simulink model "SWC_CGW_type"  (R2021b)
settings: Solver=FixedStepDiscrete  StartTime=0.0  StopTime=10.0  RelTol=1e-3
settings Model: DataDictionary=APPTypes.sldd  Creator=FVT23010  LastModifiedBy=FVT23010
settings DataIOCC: SaveFormat=StructureWithTime
settings OptimizationCC: DefaultParameterBehavior=Inlined  EnhancedBackFolding=on  PassReuseOutputArgsAs=Individual arguments  ZeroExternalMemoryAtStartup=off  ZeroInternalMemoryAtStartup=off  OptimizeBlockOrder=speed  DifferentSizesBufferReuse=on  OptimizationCustomize=off  EfficientTunableParamExpr=on
settings DebuggingCC: ParameterTunabilityLossMsg=error
settings HardwareCC: ProdBitPerPointer=32  ProdBitPerSizeT=32  ProdBitPerPtrDiffT=32  ProdLargestAtomicInteger=Long  ProdLargestAtomicFloat=Double  ProdWordSize=32  ProdLongLongMode=on  ProdHWDeviceType=ARM Compatible->ARM Cortex-M
settings ModelReferenceCC: ModelReferenceNumInstancesAllowed=Single
settings SFSimCC: MATLABDynamicMemAlloc=off
settings RTWCC: Description=AUTOSAR  SystemTargetFile=autosar.tlc  GenCodeOnly=on  TemplateMakefile=ert_default_tmf  PortableWordSizes=on
settings CodeAppCC: ForceParamTrailComments=on  IgnoreCustomStorageClasses=off  OperatorAnnotations=on  SimulinkDataObjDesc=on  SFDataObjDesc=on  InsertBlockDesc=on
settings STFCustomTargetCC: TargetLangStandard=C99 (ISO)  MultiwordLength=256  ParMdlRefBuildCompliant=on  CompOptLevelCompliant=on  IncludeMdlTerminateFcn=off  CombineOutputUpdateFcns=on  SuppressErrorStatus=on  ERTCustomFileBanners=on  SupportNonFinite=off  SupportComplex=off  SupportContinuousTime=off  SupportNonInlinedSFcns=off  RemoveResetFunc=on  MATLABClassNameForMDSCustomization=Simulink.SoftwareTarget.ERTCustomization  AutosarCompliant=on  GRTInterface=off  UseToolchainInfoCompliant=on  LookupTableObjectStructAxisOrder=2,1,3,4,...  LUTObjectStructOrderEvenSpacing=Size,Table,Breakpoints  SystemTargetFile=autosar.tlc
settings ERTTargetCC: TargetLangStandard=C99 (ISO)  ConcurrentExecutionCompliant=off  IncludeMdlTerminateFcn=off  SuppressErrorStatus=on  SupportNonFinite=off  SupportComplex=off  ModelStepFunctionPrototypeControlCompliant=off  CPPClassGenCompliant=off  AutosarCompliant=on  LookupTableObjectStructAxisOrder=2,1,3,4,...  LUTObjectStructOrderEvenSpacing=Size,Table,Breakpoints  GenerateASAP2=on  InlinedParameterPlacement=NonHierarchical  ERTCustomFileTemplate=example_file_process.tlc  ConvertIfToSwitch=off  SuppressUnreachableDefaultCases=off  BooleanTrueId=true_MatlabRTW  BooleanFalseId=false_MatlabRTW

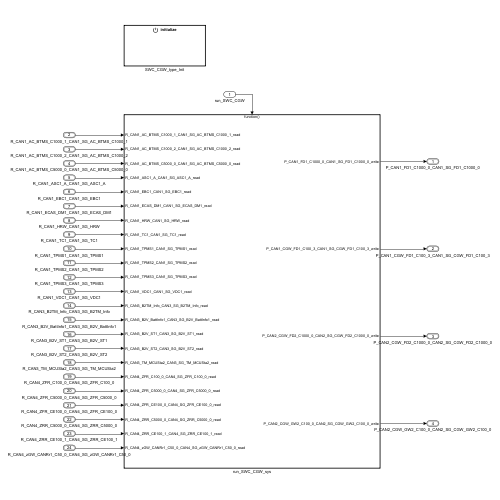
[thumbnail: Simulink's stored preview of the top-level diagram]
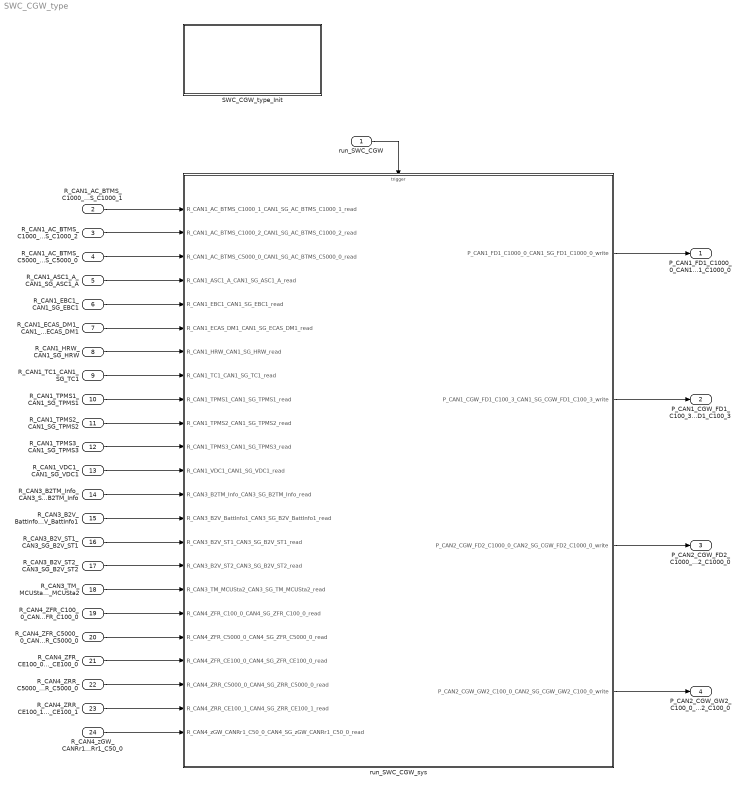
== system SWC_CGW_type ==
  run_SWC_CGW : Inport  OutputFunctionCall=on
  R_CAN1_AC_BTMS_C1000_1_CAN1_SG_AC_BTMS_C1000_1 : Inport  Port=2  OutDataTypeStr=Bus: DT_CAN1_SG_AC_BTMS_C1000_1  PortDimensions=1  BusOutputAsStruct=on
  R_CAN1_AC_BTMS_C1000_2_CAN1_SG_AC_BTMS_C1000_2 : Inport  Port=3  OutDataTypeStr=Bus: DT_CAN1_SG_AC_BTMS_C1000_2  PortDimensions=1  BusOutputAsStruct=on
  R_CAN1_AC_BTMS_C5000_0_CAN1_SG_AC_BTMS_C5000_0 : Inport  Port=4  OutDataTypeStr=Bus: DT_CAN1_SG_AC_BTMS_C5000_0  PortDimensions=1  BusOutputAsStruct=on
  R_CAN1_ASC1_A_CAN1_SG_ASC1_A : Inport  Port=5  OutDataTypeStr=Bus: DT_CAN1_SG_ASC1_A  PortDimensions=1  BusOutputAsStruct=on
  R_CAN1_EBC1_CAN1_SG_EBC1 : Inport  Port=6  OutDataTypeStr=Bus: DT_CAN1_SG_EBC1  PortDimensions=1  BusOutputAsStruct=on
  R_CAN1_ECAS_DM1_CAN1_SG_ECAS_DM1 : Inport  Port=7  OutDataTypeStr=Bus: DT_CAN1_SG_ECAS_DM1  PortDimensions=1  BusOutputAsStruct=on
  R_CAN1_HRW_CAN1_SG_HRW : Inport  Port=8  OutDataTypeStr=Bus: DT_CAN1_SG_HRW  PortDimensions=1  BusOutputAsStruct=on
  R_CAN1_TC1_CAN1_SG_TC1 : Inport  Port=9  OutDataTypeStr=Bus: DT_CAN1_SG_TC1  PortDimensions=1  BusOutputAsStruct=on
  R_CAN1_TPMS1_CAN1_SG_TPMS1 : Inport  Port=10  OutDataTypeStr=Bus: DT_CAN1_SG_TPMS1  PortDimensions=1  BusOutputAsStruct=on
  R_CAN1_TPMS2_CAN1_SG_TPMS2 : Inport  Port=11  OutDataTypeStr=Bus: DT_CAN1_SG_TPMS2  PortDimensions=1  BusOutputAsStruct=on
  R_CAN1_TPMS3_CAN1_SG_TPMS3 : Inport  Port=12  OutDataTypeStr=Bus: DT_CAN1_SG_TPMS3  PortDimensions=1  BusOutputAsStruct=on
  R_CAN1_VDC1_CAN1_SG_VDC1 : Inport  Port=13  OutDataTypeStr=Bus: DT_CAN1_SG_VDC1  PortDimensions=1  BusOutputAsStruct=on
  R_CAN3_B2TM_Info_CAN3_SG_B2TM_Info : Inport  Port=14  OutDataTypeStr=Bus: DT_CAN3_SG_B2TM_Info  PortDimensions=1  BusOutputAsStruct=on
  R_CAN3_B2V_BattInfo1_CAN3_SG_B2V_BattInfo1 : Inport  Port=15  OutDataTypeStr=Bus: DT_CAN3_SG_B2V_BattInfo1  PortDimensions=1  BusOutputAsStruct=on
  R_CAN3_B2V_ST1_CAN3_SG_B2V_ST1 : Inport  Port=16  OutDataTypeStr=Bus: DT_CAN3_SG_B2V_ST1  PortDimensions=1  BusOutputAsStruct=on
  R_CAN3_B2V_ST2_CAN3_SG_B2V_ST2 : Inport  Port=17  OutDataTypeStr=Bus: DT_CAN3_SG_B2V_ST2  PortDimensions=1  BusOutputAsStruct=on
  R_CAN3_TM_MCUSta2_CAN3_SG_TM_MCUSta2 : Inport  Port=18  OutDataTypeStr=Bus: DT_CAN3_SG_TM_MCUSta2  PortDimensions=1  BusOutputAsStruct=on
  R_CAN4_ZFR_C100_0_CAN4_SG_ZFR_C100_0 : Inport  Port=19  OutDataTypeStr=Bus: DT_CAN4_SG_ZFR_C100_0  PortDimensions=1  BusOutputAsStruct=on
  R_CAN4_ZFR_C5000_0_CAN4_SG_ZFR_C5000_0 : Inport  Port=20  OutDataTypeStr=Bus: DT_CAN4_SG_ZFR_C5000_0  PortDimensions=1  BusOutputAsStruct=on
  R_CAN4_ZFR_CE100_0_CAN4_SG_ZFR_CE100_0 : Inport  Port=21  OutDataTypeStr=Bus: DT_CAN4_SG_ZFR_CE100_0  PortDimensions=1  BusOutputAsStruct=on
  R_CAN4_ZRR_C5000_0_CAN4_SG_ZRR_C5000_0 : Inport  Port=22  OutDataTypeStr=Bus: DT_CAN4_SG_ZRR_C5000_0  PortDimensions=1  BusOutputAsStruct=on
  R_CAN4_ZRR_CE100_1_CAN4_SG_ZRR_CE100_1 : Inport  Port=23  OutDataTypeStr=Bus: DT_CAN4_SG_ZRR_CE100_1  PortDimensions=1  BusOutputAsStruct=on
  R_CAN4_zGW_CANRr1_C50_0_CAN4_SG_zGW_CANRr1_C50_0 : Inport  Port=24  OutDataTypeStr=Bus: DT_CAN4_SG_zGW_CANRr1_C50_0  PortDimensions=1  BusOutputAsStruct=on
  SWC_CGW_type_Init : Subsystem
  run_SWC_CGW_sys : Subsystem
  P_CAN1_FD1_C1000_0_CAN1_SG_FD1_C1000_0 : Outport  OutDataTypeStr=Bus: DT_CAN1_SG_FD1_C1000_0  PortDimensions=1  BusOutputAsStruct=on
  P_CAN1_CGW_FD1_C100_3_CAN1_SG_CGW_FD1_C100_3 : Outport  Port=2  OutDataTypeStr=Bus: DT_CAN1_SG_CGW_FD1_C100_3  PortDimensions=1  BusOutputAsStruct=on
  P_CAN2_CGW_FD2_C1000_0_CAN2_SG_CGW_FD2_C1000_0 : Outport  Port=3  OutDataTypeStr=Bus: DT_CAN2_SG_CGW_FD2_C1000_0  PortDimensions=1  BusOutputAsStruct=on
  P_CAN2_CGW_GW2_C100_0_CAN2_SG_CGW_GW2_C100_0 : Outport  Port=4  OutDataTypeStr=Bus: DT_CAN2_SG_CGW_GW2_C100_0  PortDimensions=1  BusOutputAsStruct=on
  wires:
  R_CAN1_AC_BTMS_C1000_1_CAN1_SG_AC_BTMS_C1000_1/1 -> run_SWC_CGW_sys/1(R_CAN1_AC_BTMS_C1000_1_CAN1_SG_AC_BTMS_C1000_1_read)
  R_CAN1_AC_BTMS_C1000_2_CAN1_SG_AC_BTMS_C1000_2/1 -> run_SWC_CGW_sys/2(R_CAN1_AC_BTMS_C1000_2_CAN1_SG_AC_BTMS_C1000_2_read)
  R_CAN1_AC_BTMS_C5000_0_CAN1_SG_AC_BTMS_C5000_0/1 -> run_SWC_CGW_sys/3(R_CAN1_AC_BTMS_C5000_0_CAN1_SG_AC_BTMS_C5000_0_read)
  R_CAN1_ASC1_A_CAN1_SG_ASC1_A/1 -> run_SWC_CGW_sys/4(R_CAN1_ASC1_A_CAN1_SG_ASC1_A_read)
  R_CAN1_EBC1_CAN1_SG_EBC1/1 -> run_SWC_CGW_sys/5(R_CAN1_EBC1_CAN1_SG_EBC1_read)
  R_CAN1_ECAS_DM1_CAN1_SG_ECAS_DM1/1 -> run_SWC_CGW_sys/6(R_CAN1_ECAS_DM1_CAN1_SG_ECAS_DM1_read)
  R_CAN1_HRW_CAN1_SG_HRW/1 -> run_SWC_CGW_sys/7(R_CAN1_HRW_CAN1_SG_HRW_read)
  R_CAN1_TC1_CAN1_SG_TC1/1 -> run_SWC_CGW_sys/8(R_CAN1_TC1_CAN1_SG_TC1_read)
  R_CAN1_TPMS1_CAN1_SG_TPMS1/1 -> run_SWC_CGW_sys/9(R_CAN1_TPMS1_CAN1_SG_TPMS1_read)
  R_CAN1_TPMS2_CAN1_SG_TPMS2/1 -> run_SWC_CGW_sys/10(R_CAN1_TPMS2_CAN1_SG_TPMS2_read)
  R_CAN1_TPMS3_CAN1_SG_TPMS3/1 -> run_SWC_CGW_sys/11(R_CAN1_TPMS3_CAN1_SG_TPMS3_read)
  R_CAN1_VDC1_CAN1_SG_VDC1/1 -> run_SWC_CGW_sys/12(R_CAN1_VDC1_CAN1_SG_VDC1_read)
  R_CAN3_B2TM_Info_CAN3_SG_B2TM_Info/1 -> run_SWC_CGW_sys/13(R_CAN3_B2TM_Info_CAN3_SG_B2TM_Info_read)
  R_CAN3_B2V_BattInfo1_CAN3_SG_B2V_BattInfo1/1 -> run_SWC_CGW_sys/14(R_CAN3_B2V_BattInfo1_CAN3_SG_B2V_BattInfo1_read)
  R_CAN3_B2V_ST1_CAN3_SG_B2V_ST1/1 -> run_SWC_CGW_sys/15(R_CAN3_B2V_ST1_CAN3_SG_B2V_ST1_read)
  R_CAN3_B2V_ST2_CAN3_SG_B2V_ST2/1 -> run_SWC_CGW_sys/16(R_CAN3_B2V_ST2_CAN3_SG_B2V_ST2_read)
  R_CAN3_TM_MCUSta2_CAN3_SG_TM_MCUSta2/1 -> run_SWC_CGW_sys/17(R_CAN3_TM_MCUSta2_CAN3_SG_TM_MCUSta2_read)
  R_CAN4_ZFR_C100_0_CAN4_SG_ZFR_C100_0/1 -> run_SWC_CGW_sys/18(R_CAN4_ZFR_C100_0_CAN4_SG_ZFR_C100_0_read)
  R_CAN4_ZFR_C5000_0_CAN4_SG_ZFR_C5000_0/1 -> run_SWC_CGW_sys/19(R_CAN4_ZFR_C5000_0_CAN4_SG_ZFR_C5000_0_read)
  R_CAN4_ZFR_CE100_0_CAN4_SG_ZFR_CE100_0/1 -> run_SWC_CGW_sys/20(R_CAN4_ZFR_CE100_0_CAN4_SG_ZFR_CE100_0_read)
  R_CAN4_ZRR_C5000_0_CAN4_SG_ZRR_C5000_0/1 -> run_SWC_CGW_sys/21(R_CAN4_ZRR_C5000_0_CAN4_SG_ZRR_C5000_0_read)
  R_CAN4_ZRR_CE100_1_CAN4_SG_ZRR_CE100_1/1 -> run_SWC_CGW_sys/22(R_CAN4_ZRR_CE100_1_CAN4_SG_ZRR_CE100_1_read)
  R_CAN4_zGW_CANRr1_C50_0_CAN4_SG_zGW_CANRr1_C50_0/1 -> run_SWC_CGW_sys/23(R_CAN4_zGW_CANRr1_C50_0_CAN4_SG_zGW_CANRr1_C50_0_read)
  run_SWC_CGW_sys/1(P_CAN1_FD1_C1000_0_CAN1_SG_FD1_C1000_0_write) -> P_CAN1_FD1_C1000_0_CAN1_SG_FD1_C1000_0/1
  run_SWC_CGW_sys/2(P_CAN1_CGW_FD1_C100_3_CAN1_SG_CGW_FD1_C100_3_write) -> P_CAN1_CGW_FD1_C100_3_CAN1_SG_CGW_FD1_C100_3/1
  run_SWC_CGW_sys/3(P_CAN2_CGW_FD2_C1000_0_CAN2_SG_CGW_FD2_C1000_0_write) -> P_CAN2_CGW_FD2_C1000_0_CAN2_SG_CGW_FD2_C1000_0/1
  run_SWC_CGW_sys/4(P_CAN2_CGW_GW2_C100_0_CAN2_SG_CGW_GW2_C100_0_write) -> P_CAN2_CGW_GW2_C100_0_CAN2_SG_CGW_GW2_C100_0/1
  run_SWC_CGW/1 -> run_SWC_CGW_sys/Trigger

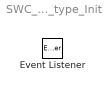
== system SWC_CGW_type/SWC_CGW_type_Init ==
  Event Listener : EventListener  EventName=reset

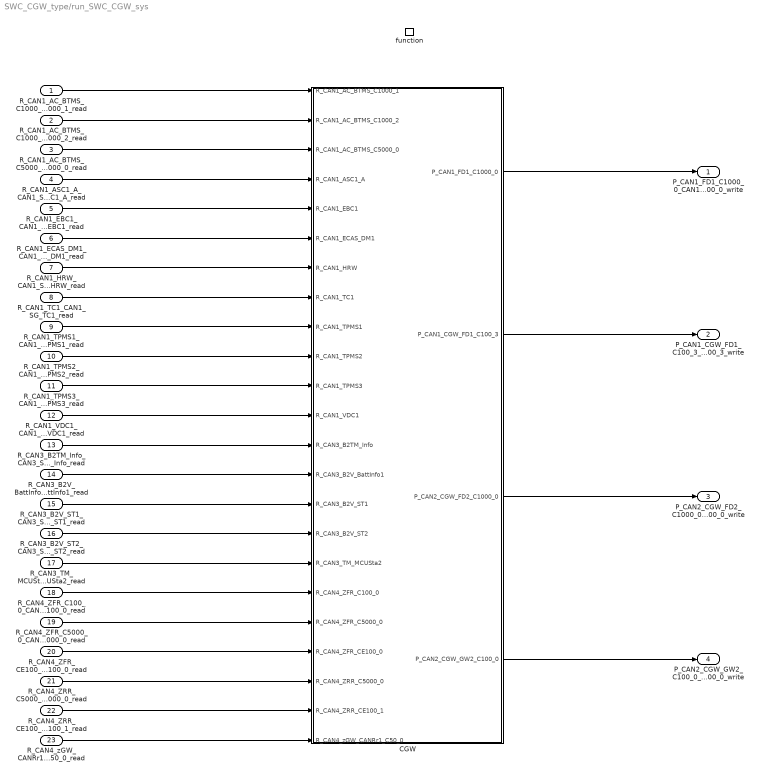
== system SWC_CGW_type/run_SWC_CGW_sys ==
  R_CAN1_AC_BTMS_C1000_1_CAN1_SG_AC_BTMS_C1000_1_read : Inport
  R_CAN1_AC_BTMS_C1000_2_CAN1_SG_AC_BTMS_C1000_2_read : Inport  Port=2
  R_CAN1_AC_BTMS_C5000_0_CAN1_SG_AC_BTMS_C5000_0_read : Inport  Port=3
  R_CAN1_ASC1_A_CAN1_SG_ASC1_A_read : Inport  Port=4
  R_CAN1_EBC1_CAN1_SG_EBC1_read : Inport  Port=5
  R_CAN1_ECAS_DM1_CAN1_SG_ECAS_DM1_read : Inport  Port=6
  R_CAN1_HRW_CAN1_SG_HRW_read : Inport  Port=7
  R_CAN1_TC1_CAN1_SG_TC1_read : Inport  Port=8
  R_CAN1_TPMS1_CAN1_SG_TPMS1_read : Inport  Port=9
  R_CAN1_TPMS2_CAN1_SG_TPMS2_read : Inport  Port=10
  R_CAN1_TPMS3_CAN1_SG_TPMS3_read : Inport  Port=11
  R_CAN1_VDC1_CAN1_SG_VDC1_read : Inport  Port=12
  R_CAN3_B2TM_Info_CAN3_SG_B2TM_Info_read : Inport  Port=13
  R_CAN3_B2V_BattInfo1_CAN3_SG_B2V_BattInfo1_read : Inport  Port=14
  R_CAN3_B2V_ST1_CAN3_SG_B2V_ST1_read : Inport  Port=15
  R_CAN3_B2V_ST2_CAN3_SG_B2V_ST2_read : Inport  Port=16
  R_CAN3_TM_MCUSta2_CAN3_SG_TM_MCUSta2_read : Inport  Port=17
  R_CAN4_ZFR_C100_0_CAN4_SG_ZFR_C100_0_read : Inport  Port=18
  R_CAN4_ZFR_C5000_0_CAN4_SG_ZFR_C5000_0_read : Inport  Port=19
  R_CAN4_ZFR_CE100_0_CAN4_SG_ZFR_CE100_0_read : Inport  Port=20
  R_CAN4_ZRR_C5000_0_CAN4_SG_ZRR_C5000_0_read : Inport  Port=21
  R_CAN4_ZRR_CE100_1_CAN4_SG_ZRR_CE100_1_read : Inport  Port=22
  R_CAN4_zGW_CANRr1_C50_0_CAN4_SG_zGW_CANRr1_C50_0_read : Inport  Port=23
  function : TriggerPort  TriggerType=function-call  VariantControl=(inherit)
  CGW : Subsystem
  P_CAN1_FD1_C1000_0_CAN1_SG_FD1_C1000_0_write : Outport
  P_CAN1_CGW_FD1_C100_3_CAN1_SG_CGW_FD1_C100_3_write : Outport  Port=2
  P_CAN2_CGW_FD2_C1000_0_CAN2_SG_CGW_FD2_C1000_0_write : Outport  Port=3
  P_CAN2_CGW_GW2_C100_0_CAN2_SG_CGW_GW2_C100_0_write : Outport  Port=4
  wires:
  R_CAN3_TM_MCUSta2_CAN3_SG_TM_MCUSta2_read/1 -> CGW/17(R_CAN3_TM_MCUSta2)
  R_CAN3_B2V_ST1_CAN3_SG_B2V_ST1_read/1 -> CGW/15(R_CAN3_B2V_ST1)
  R_CAN3_B2V_ST2_CAN3_SG_B2V_ST2_read/1 -> CGW/16(R_CAN3_B2V_ST2)
  R_CAN4_ZFR_C100_0_CAN4_SG_ZFR_C100_0_read/1 -> CGW/18(R_CAN4_ZFR_C100_0)
  R_CAN4_ZFR_C5000_0_CAN4_SG_ZFR_C5000_0_read/1 -> CGW/19(R_CAN4_ZFR_C5000_0)
  R_CAN3_B2TM_Info_CAN3_SG_B2TM_Info_read/1 -> CGW/13(R_CAN3_B2TM_Info)
  R_CAN3_B2V_BattInfo1_CAN3_SG_B2V_BattInfo1_read/1 -> CGW/14(R_CAN3_B2V_BattInfo1)
  R_CAN4_ZFR_CE100_0_CAN4_SG_ZFR_CE100_0_read/1 -> CGW/20(R_CAN4_ZFR_CE100_0)
  R_CAN4_ZRR_C5000_0_CAN4_SG_ZRR_C5000_0_read/1 -> CGW/21(R_CAN4_ZRR_C5000_0)
  R_CAN1_VDC1_CAN1_SG_VDC1_read/1 -> CGW/12(R_CAN1_VDC1)
  R_CAN4_ZRR_CE100_1_CAN4_SG_ZRR_CE100_1_read/1 -> CGW/22(R_CAN4_ZRR_CE100_1)
  R_CAN1_TPMS2_CAN1_SG_TPMS2_read/1 -> CGW/10(R_CAN1_TPMS2)
  R_CAN1_TPMS3_CAN1_SG_TPMS3_read/1 -> CGW/11(R_CAN1_TPMS3)
  R_CAN4_zGW_CANRr1_C50_0_CAN4_SG_zGW_CANRr1_C50_0_read/1 -> CGW/23(R_CAN4_zGW_CANRr1_C50_0)
  R_CAN1_TC1_CAN1_SG_TC1_read/1 -> CGW/8(R_CAN1_TC1)
  R_CAN1_TPMS1_CAN1_SG_TPMS1_read/1 -> CGW/9(R_CAN1_TPMS1)
  R_CAN1_HRW_CAN1_SG_HRW_read/1 -> CGW/7(R_CAN1_HRW)
  R_CAN1_EBC1_CAN1_SG_EBC1_read/1 -> CGW/5(R_CAN1_EBC1)
  R_CAN1_ECAS_DM1_CAN1_SG_ECAS_DM1_read/1 -> CGW/6(R_CAN1_ECAS_DM1)
  R_CAN1_AC_BTMS_C5000_0_CAN1_SG_AC_BTMS_C5000_0_read/1 -> CGW/3(R_CAN1_AC_BTMS_C5000_0)
  R_CAN1_ASC1_A_CAN1_SG_ASC1_A_read/1 -> CGW/4(R_CAN1_ASC1_A)
  R_CAN1_AC_BTMS_C1000_2_CAN1_SG_AC_BTMS_C1000_2_read/1 -> CGW/2(R_CAN1_AC_BTMS_C1000_2)
  R_CAN1_AC_BTMS_C1000_1_CAN1_SG_AC_BTMS_C1000_1_read/1 -> CGW/1(R_CAN1_AC_BTMS_C1000_1)
  CGW/1(P_CAN1_FD1_C1000_0) -> P_CAN1_FD1_C1000_0_CAN1_SG_FD1_C1000_0_write/1
  CGW/2(P_CAN1_CGW_FD1_C100_3) -> P_CAN1_CGW_FD1_C100_3_CAN1_SG_CGW_FD1_C100_3_write/1
  CGW/3(P_CAN2_CGW_FD2_C1000_0) -> P_CAN2_CGW_FD2_C1000_0_CAN2_SG_CGW_FD2_C1000_0_write/1
  CGW/4(P_CAN2_CGW_GW2_C100_0) -> P_CAN2_CGW_GW2_C100_0_CAN2_SG_CGW_GW2_C100_0_write/1

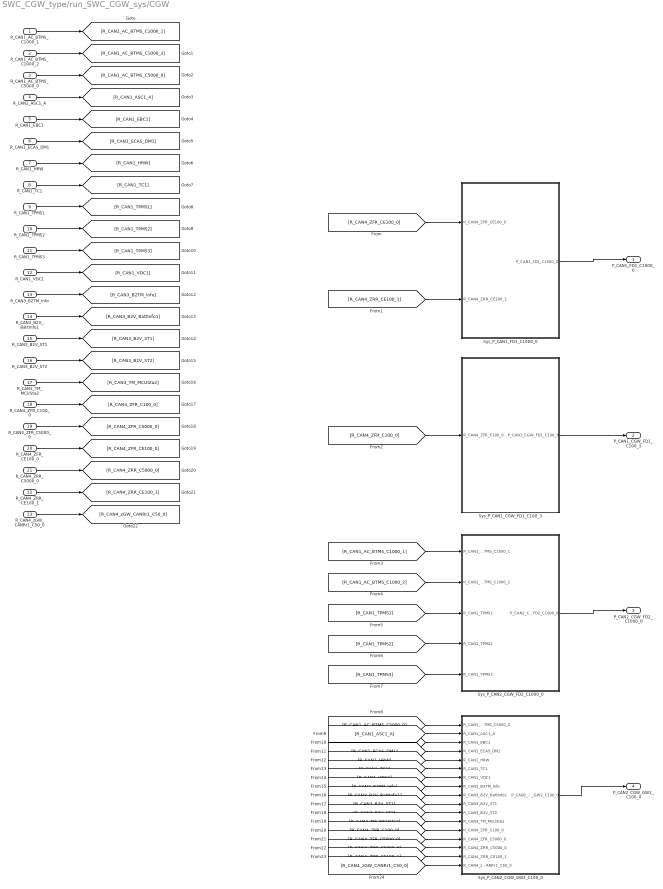
== system SWC_CGW_type/run_SWC_CGW_sys/CGW ==
  R_CAN1_AC_BTMS_C1000_1 : Inport
  R_CAN1_AC_BTMS_C1000_2 : Inport  Port=2
  R_CAN1_AC_BTMS_C5000_0 : Inport  Port=3
  R_CAN1_ASC1_A : Inport  Port=4
  R_CAN1_EBC1 : Inport  Port=5
  R_CAN1_ECAS_DM1 : Inport  Port=6
  R_CAN1_HRW : Inport  Port=7
  R_CAN1_TC1 : Inport  Port=8
  R_CAN1_TPMS1 : Inport  Port=9
  R_CAN1_TPMS2 : Inport  Port=10
  R_CAN1_TPMS3 : Inport  Port=11
  R_CAN1_VDC1 : Inport  Port=12
  R_CAN3_B2TM_Info : Inport  Port=13
  R_CAN3_B2V_BattInfo1 : Inport  Port=14
  R_CAN3_B2V_ST1 : Inport  Port=15
  R_CAN3_B2V_ST2 : Inport  Port=16
  R_CAN3_TM_MCUSta2 : Inport  Port=17
  R_CAN4_ZFR_C100_0 : Inport  Port=18
  R_CAN4_ZFR_C5000_0 : Inport  Port=19
  R_CAN4_ZFR_CE100_0 : Inport  Port=20
  R_CAN4_ZRR_C5000_0 : Inport  Port=21
  R_CAN4_ZRR_CE100_1 : Inport  Port=22
  R_CAN4_zGW_CANRr1_C50_0 : Inport  Port=23
  Sys_P_CAN1_CGW_FD1_C100_3 : Subsystem
  Sys_P_CAN1_FD1_C1000_0 : Subsystem
  Sys_P_CAN2_CGW_FD2_C1000_0 : Subsystem
  Sys_P_CAN2_CGW_GW2_C100_0 : Subsystem
  P_CAN1_FD1_C1000_0 : Outport
  P_CAN1_CGW_FD1_C100_3 : Outport  Port=2
  P_CAN2_CGW_FD2_C1000_0 : Outport  Port=3
  P_CAN2_CGW_GW2_C100_0 : Outport  Port=4
  wires:
  R_CAN1_AC_BTMS_C1000_1/1 -> [R_CAN1_AC_BTMS_C1000_1]
  R_CAN1_AC_BTMS_C1000_2/1 -> [R_CAN1_AC_BTMS_C1000_2]
  R_CAN1_AC_BTMS_C5000_0/1 -> [R_CAN1_AC_BTMS_C5000_0]
  R_CAN1_ASC1_A/1 -> [R_CAN1_ASC1_A]
  R_CAN1_EBC1/1 -> [R_CAN1_EBC1]
  R_CAN1_ECAS_DM1/1 -> [R_CAN1_ECAS_DM1]
  R_CAN1_HRW/1 -> [R_CAN1_HRW]
  R_CAN1_TC1/1 -> [R_CAN1_TC1]
  R_CAN1_TPMS1/1 -> [R_CAN1_TPMS1]
  R_CAN1_TPMS2/1 -> [R_CAN1_TPMS2]
  R_CAN1_TPMS3/1 -> [R_CAN1_TPMS3]
  R_CAN1_VDC1/1 -> [R_CAN1_VDC1]
  R_CAN3_B2TM_Info/1 -> [R_CAN3_B2TM_Info]
  R_CAN3_B2V_BattInfo1/1 -> [R_CAN3_B2V_BattInfo1]
  R_CAN3_B2V_ST1/1 -> [R_CAN3_B2V_ST1]
  R_CAN3_B2V_ST2/1 -> [R_CAN3_B2V_ST2]
  R_CAN3_TM_MCUSta2/1 -> [R_CAN3_TM_MCUSta2]
  R_CAN4_ZFR_C100_0/1 -> [R_CAN4_ZFR_C100_0]
  R_CAN4_ZFR_C5000_0/1 -> [R_CAN4_ZFR_C5000_0]
  R_CAN4_ZFR_CE100_0/1 -> [R_CAN4_ZFR_CE100_0]
  R_CAN4_ZRR_C5000_0/1 -> [R_CAN4_ZRR_C5000_0]
  R_CAN4_ZRR_CE100_1/1 -> [R_CAN4_ZRR_CE100_1]
  R_CAN4_zGW_CANRr1_C50_0/1 -> [R_CAN4_zGW_CANRr1_C50_0]
  Sys_P_CAN1_FD1_C1000_0/1(P_CAN1_FD1_C1000_0) -> P_CAN1_FD1_C1000_0/1
  Sys_P_CAN1_CGW_FD1_C100_3/1(P_CAN1_CGW_FD1_C100_3) -> P_CAN1_CGW_FD1_C100_3/1
  Sys_P_CAN2_CGW_FD2_C1000_0/1(P_CAN2_CGW_FD2_C1000_0) -> P_CAN2_CGW_FD2_C1000_0/1
  Sys_P_CAN2_CGW_GW2_C100_0/1(P_CAN2_CGW_GW2_C100_0) -> P_CAN2_CGW_GW2_C100_0/1
  [R_CAN4_ZFR_CE100_0] -> Sys_P_CAN1_FD1_C1000_0/1(R_CAN4_ZFR_CE100_0)
  [R_CAN4_ZRR_CE100_1] -> Sys_P_CAN1_FD1_C1000_0/2(R_CAN4_ZRR_CE100_1)
  [R_CAN4_ZFR_C100_0] -> Sys_P_CAN1_CGW_FD1_C100_3/1(R_CAN4_ZFR_C100_0)
  [R_CAN1_AC_BTMS_C1000_1] -> Sys_P_CAN2_CGW_FD2_C1000_0/1(R_CAN1_AC_BTMS_C1000_1)
  [R_CAN1_AC_BTMS_C1000_2] -> Sys_P_CAN2_CGW_FD2_C1000_0/2(R_CAN1_AC_BTMS_C1000_2)
  [R_CAN1_TPMS1] -> Sys_P_CAN2_CGW_FD2_C1000_0/3(R_CAN1_TPMS1)
  [R_CAN1_TPMS2] -> Sys_P_CAN2_CGW_FD2_C1000_0/4(R_CAN1_TPMS2)
  [R_CAN1_TPMS3] -> Sys_P_CAN2_CGW_FD2_C1000_0/5(R_CAN1_TPMS3)
  [R_CAN1_AC_BTMS_C5000_0] -> Sys_P_CAN2_CGW_GW2_C100_0/1(R_CAN1_AC_BTMS_C5000_0)
  [R_CAN1_ASC1_A] -> Sys_P_CAN2_CGW_GW2_C100_0/2(R_CAN1_ASC1_A)
  [R_CAN1_EBC1] -> Sys_P_CAN2_CGW_GW2_C100_0/3(R_CAN1_EBC1)
  [R_CAN1_ECAS_DM1] -> Sys_P_CAN2_CGW_GW2_C100_0/4(R_CAN1_ECAS_DM1)
  [R_CAN1_HRW] -> Sys_P_CAN2_CGW_GW2_C100_0/5(R_CAN1_HRW)
  [R_CAN1_TC1] -> Sys_P_CAN2_CGW_GW2_C100_0/6(R_CAN1_TC1)
  [R_CAN1_VDC1] -> Sys_P_CAN2_CGW_GW2_C100_0/7(R_CAN1_VDC1)
  [R_CAN3_B2TM_Info] -> Sys_P_CAN2_CGW_GW2_C100_0/8(R_CAN3_B2TM_Info)
  [R_CAN3_B2V_BattInfo1] -> Sys_P_CAN2_CGW_GW2_C100_0/9(R_CAN3_B2V_BattInfo1)
  [R_CAN3_B2V_ST1] -> Sys_P_CAN2_CGW_GW2_C100_0/10(R_CAN3_B2V_ST1)
  [R_CAN3_B2V_ST2] -> Sys_P_CAN2_CGW_GW2_C100_0/11(R_CAN3_B2V_ST2)
  [R_CAN3_TM_MCUSta2] -> Sys_P_CAN2_CGW_GW2_C100_0/12(R_CAN3_TM_MCUSta2)
  [R_CAN4_ZFR_C100_0] -> Sys_P_CAN2_CGW_GW2_C100_0/13(R_CAN4_ZFR_C100_0)
  [R_CAN4_ZFR_C5000_0] -> Sys_P_CAN2_CGW_GW2_C100_0/14(R_CAN4_ZFR_C5000_0)
  [R_CAN4_ZRR_C5000_0] -> Sys_P_CAN2_CGW_GW2_C100_0/15(R_CAN4_ZRR_C5000_0)
  [R_CAN4_ZRR_CE100_1] -> Sys_P_CAN2_CGW_GW2_C100_0/16(R_CAN4_ZRR_CE100_1)
  [R_CAN4_zGW_CANRr1_C50_0] -> Sys_P_CAN2_CGW_GW2_C100_0/17(R_CAN4_zGW_CANRr1_C50_0)

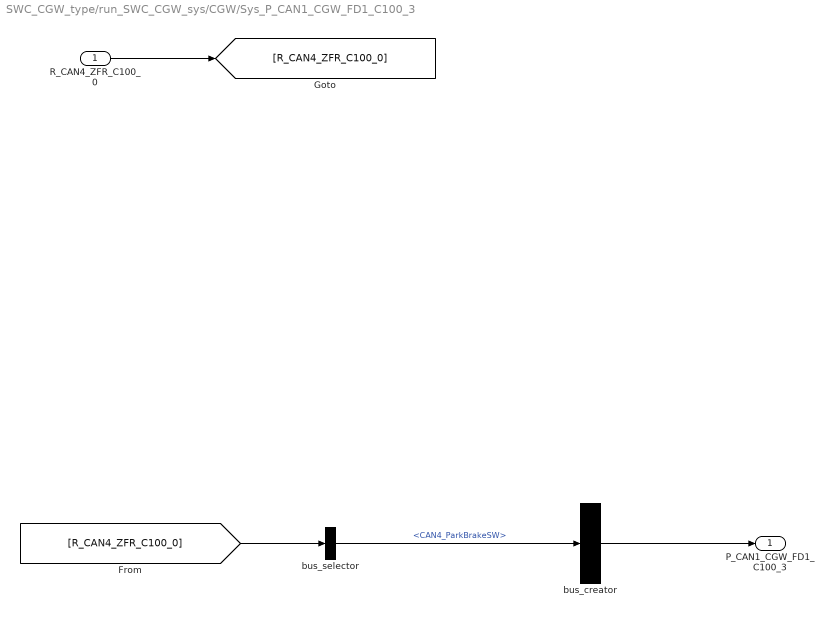
== system SWC_CGW_type/run_SWC_CGW_sys/CGW/Sys_P_CAN1_CGW_FD1_C100_3 ==
  R_CAN4_ZFR_C100_0 : Inport
  bus_creator : BusCreator  Inputs=1  OutDataTypeStr=Bus: DT_CAN1_SG_CGW_FD1_C100_3  NonVirtualBus=on
  bus_selector : BusSelector  OutputSignals=CAN4_ParkBrakeSW
  P_CAN1_CGW_FD1_C100_3 : Outport
  wires:
  bus_creator/1 -> P_CAN1_CGW_FD1_C100_3/1
  bus_selector/1 -> bus_creator/1  "<CAN4_ParkBrakeSW>"
  [R_CAN4_ZFR_C100_0] -> bus_selector/1
  R_CAN4_ZFR_C100_0/1 -> [R_CAN4_ZFR_C100_0]

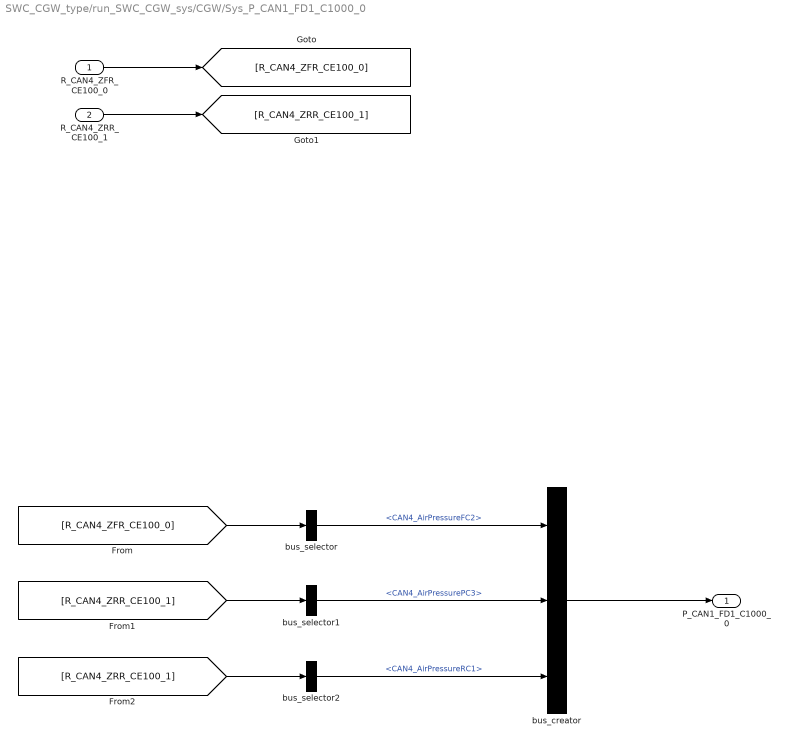
== system SWC_CGW_type/run_SWC_CGW_sys/CGW/Sys_P_CAN1_FD1_C1000_0 ==
  R_CAN4_ZFR_CE100_0 : Inport
  R_CAN4_ZRR_CE100_1 : Inport  Port=2
  bus_creator : BusCreator  Inputs=3  OutDataTypeStr=Bus: DT_CAN1_SG_FD1_C1000_0  NonVirtualBus=on
  bus_selector : BusSelector  OutputSignals=CAN4_AirPressureFC2
  bus_selector1 : BusSelector  OutputSignals=CAN4_AirPressurePC3
  bus_selector2 : BusSelector  OutputSignals=CAN4_AirPressureRC1
  P_CAN1_FD1_C1000_0 : Outport
  wires:
  bus_creator/1 -> P_CAN1_FD1_C1000_0/1
  bus_selector/1 -> bus_creator/1  "<CAN4_AirPressureFC2>"
  [R_CAN4_ZFR_CE100_0] -> bus_selector/1
  bus_selector1/1 -> bus_creator/2  "<CAN4_AirPressurePC3>"
  [R_CAN4_ZRR_CE100_1] -> bus_selector1/1
  bus_selector2/1 -> bus_creator/3  "<CAN4_AirPressureRC1>"
  [R_CAN4_ZRR_CE100_1] -> bus_selector2/1
  R_CAN4_ZFR_CE100_0/1 -> [R_CAN4_ZFR_CE100_0]
  R_CAN4_ZRR_CE100_1/1 -> [R_CAN4_ZRR_CE100_1]

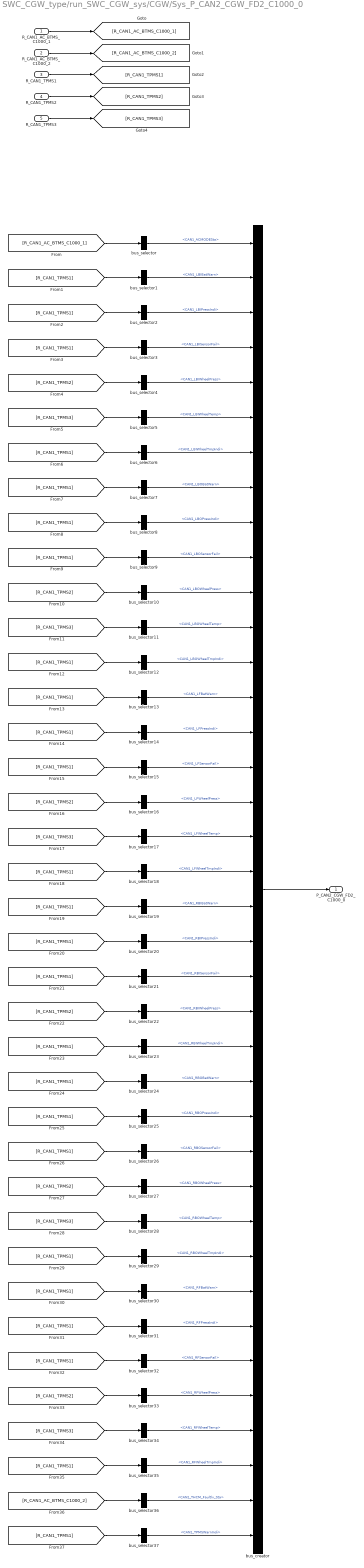
== system SWC_CGW_type/run_SWC_CGW_sys/CGW/Sys_P_CAN2_CGW_FD2_C1000_0 ==
  R_CAN1_AC_BTMS_C1000_1 : Inport
  R_CAN1_AC_BTMS_C1000_2 : Inport  Port=2
  R_CAN1_TPMS1 : Inport  Port=3
  R_CAN1_TPMS2 : Inport  Port=4
  R_CAN1_TPMS3 : Inport  Port=5
  bus_creator : BusCreator  Inputs=38  OutDataTypeStr=Bus: DT_CAN2_SG_CGW_FD2_C1000_0  NonVirtualBus=on
  bus_selector : BusSelector  OutputSignals=CAN1_ACMODESta
  bus_selector1 : BusSelector  OutputSignals=CAN1_LBIBatWarn
  bus_selector10 : BusSelector  OutputSignals=CAN1_LBOWheelPress
  bus_selector11 : BusSelector  OutputSignals=CAN1_LBOWheelTemp
  bus_selector12 : BusSelector  OutputSignals=CAN1_LBOWheelTmpIndi
  bus_selector13 : BusSelector  OutputSignals=CAN1_LFBatWarn
  bus_selector14 : BusSelector  OutputSignals=CAN1_LFPressIndi
  bus_selector15 : BusSelector  OutputSignals=CAN1_LFSensorFail
  bus_selector16 : BusSelector  OutputSignals=CAN1_LFWheelPress
  bus_selector17 : BusSelector  OutputSignals=CAN1_LFWheelTemp
  bus_selector18 : BusSelector  OutputSignals=CAN1_LFWheelTmpIndi
  bus_selector19 : BusSelector  OutputSignals=CAN1_RBIBatWarn
  bus_selector2 : BusSelector  OutputSignals=CAN1_LBIPressIndi
  bus_selector20 : BusSelector  OutputSignals=CAN1_RBIPressIndi
  bus_selector21 : BusSelector  OutputSignals=CAN1_RBISensorFail
  bus_selector22 : BusSelector  OutputSignals=CAN1_RBIWheelPress
  bus_selector23 : BusSelector  OutputSignals=CAN1_RBIWheelTmpIndi
  bus_selector24 : BusSelector  OutputSignals=CAN1_RBOBatWarn
  bus_selector25 : BusSelector  OutputSignals=CAN1_RBOPressIndi
  bus_selector26 : BusSelector  OutputSignals=CAN1_RBOSensorFail
  bus_selector27 : BusSelector  OutputSignals=CAN1_RBOWheelPress
  bus_selector28 : BusSelector  OutputSignals=CAN1_RBOWheelTemp
  bus_selector29 : BusSelector  OutputSignals=CAN1_RBOWheelTmpIndi
  bus_selector3 : BusSelector  OutputSignals=CAN1_LBISensorFail
  bus_selector30 : BusSelector  OutputSignals=CAN1_RFBatWarn
  bus_selector31 : BusSelector  OutputSignals=CAN1_RFPressIndi
  bus_selector32 : BusSelector  OutputSignals=CAN1_RFSensorFail
  bus_selector33 : BusSelector  OutputSignals=CAN1_RFWheelPress
  bus_selector34 : BusSelector  OutputSignals=CAN1_RFWheelTemp
  bus_selector35 : BusSelector  OutputSignals=CAN1_RFWheelTmpIndi
  bus_selector36 : BusSelector  OutputSignals=CAN1_THCM_Faultlv_Sta
  bus_selector37 : BusSelector  OutputSignals=CAN1_TPMSWarnIndi
  bus_selector4 : BusSelector  OutputSignals=CAN1_LBIWheelPress
  bus_selector5 : BusSelector  OutputSignals=CAN1_LBIWheelTemp
  bus_selector6 : BusSelector  OutputSignals=CAN1_LBIWheelTmpIndi
  bus_selector7 : BusSelector  OutputSignals=CAN1_LBOBatWarn
  bus_selector8 : BusSelector  OutputSignals=CAN1_LBOPressIndi
  bus_selector9 : BusSelector  OutputSignals=CAN1_LBOSensorFail
  P_CAN2_CGW_FD2_C1000_0 : Outport
  wires:
  bus_creator/1 -> P_CAN2_CGW_FD2_C1000_0/1
  bus_selector/1 -> bus_creator/1  "<CAN1_ACMODESta>"
  [R_CAN1_AC_BTMS_C1000_1] -> bus_selector/1
  bus_selector1/1 -> bus_creator/2  "<CAN1_LBIBatWarn>"
  [R_CAN1_TPMS1] -> bus_selector1/1
  bus_selector2/1 -> bus_creator/3  "<CAN1_LBIPressIndi>"
  [R_CAN1_TPMS1] -> bus_selector2/1
  bus_selector3/1 -> bus_creator/4  "<CAN1_LBISensorFail>"
  [R_CAN1_TPMS1] -> bus_selector3/1
  bus_selector4/1 -> bus_creator/5  "<CAN1_LBIWheelPress>"
  [R_CAN1_TPMS2] -> bus_selector4/1
  bus_selector5/1 -> bus_creator/6  "<CAN1_LBIWheelTemp>"
  [R_CAN1_TPMS3] -> bus_selector5/1
  bus_selector6/1 -> bus_creator/7  "<CAN1_LBIWheelTmpIndi>"
  [R_CAN1_TPMS1] -> bus_selector6/1
  bus_selector7/1 -> bus_creator/8  "<CAN1_LBOBatWarn>"
  [R_CAN1_TPMS1] -> bus_selector7/1
  bus_selector8/1 -> bus_creator/9  "<CAN1_LBOPressIndi>"
  [R_CAN1_TPMS1] -> bus_selector8/1
  bus_selector9/1 -> bus_creator/10  "<CAN1_LBOSensorFail>"
  [R_CAN1_TPMS1] -> bus_selector9/1
  bus_selector10/1 -> bus_creator/11  "<CAN1_LBOWheelPress>"
  [R_CAN1_TPMS2] -> bus_selector10/1
  bus_selector11/1 -> bus_creator/12  "<CAN1_LBOWheelTemp>"
  [R_CAN1_TPMS3] -> bus_selector11/1
  bus_selector12/1 -> bus_creator/13  "<CAN1_LBOWheelTmpIndi>"
  [R_CAN1_TPMS1] -> bus_selector12/1
  bus_selector13/1 -> bus_creator/14  "<CAN1_LFBatWarn>"
  [R_CAN1_TPMS1] -> bus_selector13/1
  bus_selector14/1 -> bus_creator/15  "<CAN1_LFPressIndi>"
  [R_CAN1_TPMS1] -> bus_selector14/1
  bus_selector15/1 -> bus_creator/16  "<CAN1_LFSensorFail>"
  [R_CAN1_TPMS1] -> bus_selector15/1
  bus_selector16/1 -> bus_creator/17  "<CAN1_LFWheelPress>"
  [R_CAN1_TPMS2] -> bus_selector16/1
  bus_selector17/1 -> bus_creator/18  "<CAN1_LFWheelTemp>"
  [R_CAN1_TPMS3] -> bus_selector17/1
  bus_selector18/1 -> bus_creator/19  "<CAN1_LFWheelTmpIndi>"
  [R_CAN1_TPMS1] -> bus_selector18/1
  bus_selector19/1 -> bus_creator/20  "<CAN1_RBIBatWarn>"
  [R_CAN1_TPMS1] -> bus_selector19/1
  bus_selector20/1 -> bus_creator/21  "<CAN1_RBIPressIndi>"
  [R_CAN1_TPMS1] -> bus_selector20/1
  bus_selector21/1 -> bus_creator/22  "<CAN1_RBISensorFail>"
  [R_CAN1_TPMS1] -> bus_selector21/1
  bus_selector22/1 -> bus_creator/23  "<CAN1_RBIWheelPress>"
  [R_CAN1_TPMS2] -> bus_selector22/1
  bus_selector23/1 -> bus_creator/24  "<CAN1_RBIWheelTmpIndi>"
  [R_CAN1_TPMS1] -> bus_selector23/1
  bus_selector24/1 -> bus_creator/25  "<CAN1_RBOBatWarn>"
  [R_CAN1_TPMS1] -> bus_selector24/1
  bus_selector25/1 -> bus_creator/26  "<CAN1_RBOPressIndi>"
  [R_CAN1_TPMS1] -> bus_selector25/1
  bus_selector26/1 -> bus_creator/27  "<CAN1_RBOSensorFail>"
  [R_CAN1_TPMS1] -> bus_selector26/1
  bus_selector27/1 -> bus_creator/28  "<CAN1_RBOWheelPress>"
  [R_CAN1_TPMS2] -> bus_selector27/1
  bus_selector28/1 -> bus_creator/29  "<CAN1_RBOWheelTemp>"
  [R_CAN1_TPMS3] -> bus_selector28/1
  bus_selector29/1 -> bus_creator/30  "<CAN1_RBOWheelTmpIndi>"
  [R_CAN1_TPMS1] -> bus_selector29/1
  bus_selector30/1 -> bus_creator/31  "<CAN1_RFBatWarn>"
  [R_CAN1_TPMS1] -> bus_selector30/1
  bus_selector31/1 -> bus_creator/32  "<CAN1_RFPressIndi>"
  [R_CAN1_TPMS1] -> bus_selector31/1
  bus_selector32/1 -> bus_creator/33  "<CAN1_RFSensorFail>"
  [R_CAN1_TPMS1] -> bus_selector32/1
  bus_selector33/1 -> bus_creator/34  "<CAN1_RFWheelPress>"
  [R_CAN1_TPMS2] -> bus_selector33/1
  bus_selector34/1 -> bus_creator/35  "<CAN1_RFWheelTemp>"
  [R_CAN1_TPMS3] -> bus_selector34/1
  bus_selector35/1 -> bus_creator/36  "<CAN1_RFWheelTmpIndi>"
  [R_CAN1_TPMS1] -> bus_selector35/1
  bus_selector36/1 -> bus_creator/37  "<CAN1_THCM_Faultlv_Sta>"
  [R_CAN1_AC_BTMS_C1000_2] -> bus_selector36/1
  bus_selector37/1 -> bus_creator/38  "<CAN1_TPMSWarnIndi>"
  [R_CAN1_TPMS1] -> bus_selector37/1
  R_CAN1_AC_BTMS_C1000_1/1 -> [R_CAN1_AC_BTMS_C1000_1]
  R_CAN1_AC_BTMS_C1000_2/1 -> [R_CAN1_AC_BTMS_C1000_2]
  R_CAN1_TPMS1/1 -> [R_CAN1_TPMS1]
  R_CAN1_TPMS2/1 -> [R_CAN1_TPMS2]
  R_CAN1_TPMS3/1 -> [R_CAN1_TPMS3]

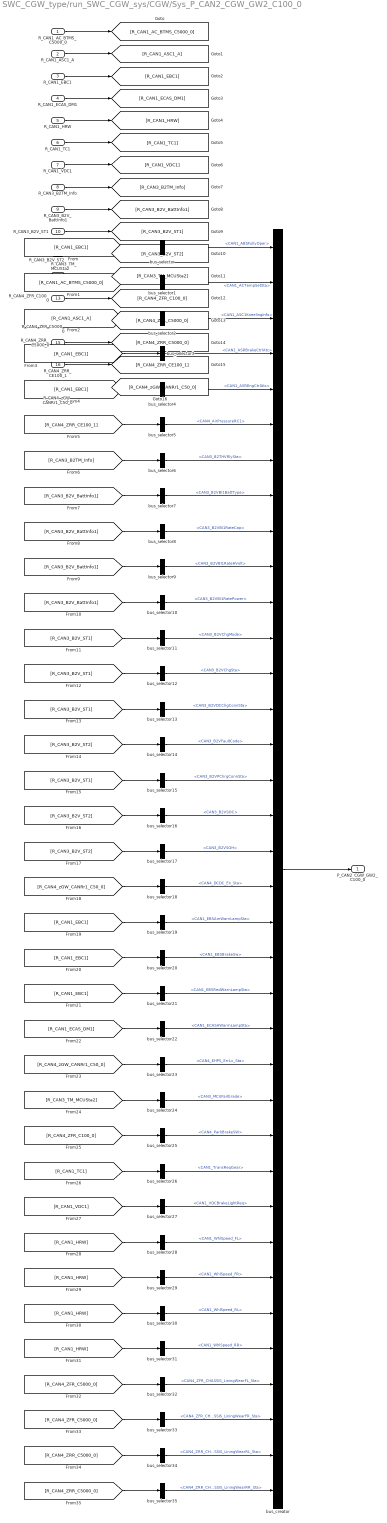
== system SWC_CGW_type/run_SWC_CGW_sys/CGW/Sys_P_CAN2_CGW_GW2_C100_0 ==
  R_CAN1_AC_BTMS_C5000_0 : Inport
  R_CAN1_ASC1_A : Inport  Port=2
  R_CAN1_EBC1 : Inport  Port=3
  R_CAN1_ECAS_DM1 : Inport  Port=4
  R_CAN1_HRW : Inport  Port=5
  R_CAN1_TC1 : Inport  Port=6
  R_CAN1_VDC1 : Inport  Port=7
  R_CAN3_B2TM_Info : Inport  Port=8
  R_CAN3_B2V_BattInfo1 : Inport  Port=9
  R_CAN3_B2V_ST1 : Inport  Port=10
  R_CAN3_B2V_ST2 : Inport  Port=11
  R_CAN3_TM_MCUSta2 : Inport  Port=12
  R_CAN4_ZFR_C100_0 : Inport  Port=13
  R_CAN4_ZFR_C5000_0 : Inport  Port=14
  R_CAN4_ZRR_C5000_0 : Inport  Port=15
  R_CAN4_ZRR_CE100_1 : Inport  Port=16
  R_CAN4_zGW_CANRr1_C50_0 : Inport  Port=17
  bus_creator : BusCreator  Inputs=36  OutDataTypeStr=Bus: DT_CAN2_SG_CGW_GW2_C100_0  NonVirtualBus=on
  bus_selector : BusSelector  OutputSignals=CAN1_ABSFullyOper
  bus_selector1 : BusSelector  OutputSignals=CAN1_ACTempSetSta
  bus_selector10 : BusSelector  OutputSignals=CAN3_B2VBI1RatePower
  bus_selector11 : BusSelector  OutputSignals=CAN3_B2VChgMode
  bus_selector12 : BusSelector  OutputSignals=CAN3_B2VChgSta
  bus_selector13 : BusSelector  OutputSignals=CAN3_B2VDCChgConnSta
  bus_selector14 : BusSelector  OutputSignals=CAN3_B2VFaultCode
  bus_selector15 : BusSelector  OutputSignals=CAN3_B2VPChrgConnSta
  bus_selector16 : BusSelector  OutputSignals=CAN3_B2VSOC
  bus_selector17 : BusSelector  OutputSignals=CAN3_B2VSOH
  bus_selector18 : BusSelector  OutputSignals=CAN4_DCDC_En_Sta
  bus_selector19 : BusSelector  OutputSignals=CAN1_EBSAmWarnLampSta
  bus_selector2 : BusSelector  OutputSignals=CAN1_ASC1KneelingInfo
  bus_selector20 : BusSelector  OutputSignals=CAN1_EBSBrakeSw
  bus_selector21 : BusSelector  OutputSignals=CAN1_EBSRedWarnLampSta
  bus_selector22 : BusSelector  OutputSignals=CAN1_ECASAWarmLampSta
  bus_selector23 : BusSelector  OutputSignals=CAN4_EHPS_ErrLv_Sta
  bus_selector24 : BusSelector  OutputSignals=CAN3_MCUFailGrade
  bus_selector25 : BusSelector  OutputSignals=CAN4_ParkBrakeSW
  bus_selector26 : BusSelector  OutputSignals=CAN1_TransReqGear
  bus_selector27 : BusSelector  OutputSignals=CAN1_VDCBrakeLightReq
  bus_selector28 : BusSelector  OutputSignals=CAN1_WhlSpeed_FL
  bus_selector29 : BusSelector  OutputSignals=CAN1_WhlSpeed_FR
  bus_selector3 : BusSelector  OutputSignals=CAN1_ASRBrakeCtrlAtc
  bus_selector30 : BusSelector  OutputSignals=CAN1_WhlSpeed_RL
  bus_selector31 : BusSelector  OutputSignals=CAN1_WhlSpeed_RR
  bus_selector32 : BusSelector  OutputSignals=CAN4_ZFR_CHASSIS_LiningWearFL_Sta
  bus_selector33 : BusSelector  OutputSignals=CAN4_ZFR_CHASSIS_LiningWearFR_Sta
  bus_selector34 : BusSelector  OutputSignals=CAN4_ZRR_CHASSIS_LiningWearRL_Sta
  bus_selector35 : BusSelector  OutputSignals=CAN4_ZRR_CHASSIS_LiningWearRR_Sta
  bus_selector4 : BusSelector  OutputSignals=CAN1_ASREngCtrlAtc
  bus_selector5 : BusSelector  OutputSignals=CAN4_AirPressureRC1
  bus_selector6 : BusSelector  OutputSignals=CAN3_B2THVRlySta
  bus_selector7 : BusSelector  OutputSignals=CAN3_B2VBI1BattType
  bus_selector8 : BusSelector  OutputSignals=CAN3_B2VBI1RateCap
  bus_selector9 : BusSelector  OutputSignals=CAN3_B2VBI1RateHVolt
  P_CAN2_CGW_GW2_C100_0 : Outport
  wires:
  bus_creator/1 -> P_CAN2_CGW_GW2_C100_0/1
  bus_selector/1 -> bus_creator/1  "<CAN1_ABSFullyOper>"
  [R_CAN1_EBC1] -> bus_selector/1
  bus_selector1/1 -> bus_creator/2  "<CAN1_ACTempSetSta>"
  [R_CAN1_AC_BTMS_C5000_0] -> bus_selector1/1
  bus_selector2/1 -> bus_creator/3  "<CAN1_ASC1KneelingInfo>"
  [R_CAN1_ASC1_A] -> bus_selector2/1
  bus_selector3/1 -> bus_creator/4  "<CAN1_ASRBrakeCtrlAtc>"
  [R_CAN1_EBC1] -> bus_selector3/1
  bus_selector4/1 -> bus_creator/5  "<CAN1_ASREngCtrlAtc>"
  [R_CAN1_EBC1] -> bus_selector4/1
  bus_selector5/1 -> bus_creator/6  "<CAN4_AirPressureRC1>"
  [R_CAN4_ZRR_CE100_1] -> bus_selector5/1
  bus_selector6/1 -> bus_creator/7  "<CAN3_B2THVRlySta>"
  [R_CAN3_B2TM_Info] -> bus_selector6/1
  bus_selector7/1 -> bus_creator/8  "<CAN3_B2VBI1BattType>"
  [R_CAN3_B2V_BattInfo1] -> bus_selector7/1
  bus_selector8/1 -> bus_creator/9  "<CAN3_B2VBI1RateCap>"
  [R_CAN3_B2V_BattInfo1] -> bus_selector8/1
  bus_selector9/1 -> bus_creator/10  "<CAN3_B2VBI1RateHVolt>"
  [R_CAN3_B2V_BattInfo1] -> bus_selector9/1
  bus_selector10/1 -> bus_creator/11  "<CAN3_B2VBI1RatePower>"
  [R_CAN3_B2V_BattInfo1] -> bus_selector10/1
  bus_selector11/1 -> bus_creator/12  "<CAN3_B2VChgMode>"
  [R_CAN3_B2V_ST1] -> bus_selector11/1
  bus_selector12/1 -> bus_creator/13  "<CAN3_B2VChgSta>"
  [R_CAN3_B2V_ST1] -> bus_selector12/1
  bus_selector13/1 -> bus_creator/14  "<CAN3_B2VDCChgConnSta>"
  [R_CAN3_B2V_ST1] -> bus_selector13/1
  bus_selector14/1 -> bus_creator/15  "<CAN3_B2VFaultCode>"
  [R_CAN3_B2V_ST2] -> bus_selector14/1
  bus_selector15/1 -> bus_creator/16  "<CAN3_B2VPChrgConnSta>"
  [R_CAN3_B2V_ST1] -> bus_selector15/1
  bus_selector16/1 -> bus_creator/17  "<CAN3_B2VSOC>"
  [R_CAN3_B2V_ST2] -> bus_selector16/1
  bus_selector17/1 -> bus_creator/18  "<CAN3_B2VSOH>"
  [R_CAN3_B2V_ST2] -> bus_selector17/1
  bus_selector18/1 -> bus_creator/19  "<CAN4_DCDC_En_Sta>"
  [R_CAN4_zGW_CANRr1_C50_0] -> bus_selector18/1
  bus_selector19/1 -> bus_creator/20  "<CAN1_EBSAmWarnLampSta>"
  [R_CAN1_EBC1] -> bus_selector19/1
  bus_selector20/1 -> bus_creator/21  "<CAN1_EBSBrakeSw>"
  [R_CAN1_EBC1] -> bus_selector20/1
  bus_selector21/1 -> bus_creator/22  "<CAN1_EBSRedWarnLampSta>"
  [R_CAN1_EBC1] -> bus_selector21/1
  bus_selector22/1 -> bus_creator/23  "<CAN1_ECASAWarmLampSta>"
  [R_CAN1_ECAS_DM1] -> bus_selector22/1
  bus_selector23/1 -> bus_creator/24  "<CAN4_EHPS_ErrLv_Sta>"
  [R_CAN4_zGW_CANRr1_C50_0] -> bus_selector23/1
  bus_selector24/1 -> bus_creator/25  "<CAN3_MCUFailGrade>"
  [R_CAN3_TM_MCUSta2] -> bus_selector24/1
  bus_selector25/1 -> bus_creator/26  "<CAN4_ParkBrakeSW>"
  [R_CAN4_ZFR_C100_0] -> bus_selector25/1
  bus_selector26/1 -> bus_creator/27  "<CAN1_TransReqGear>"
  [R_CAN1_TC1] -> bus_selector26/1
  bus_selector27/1 -> bus_creator/28  "<CAN1_VDCBrakeLightReq>"
  [R_CAN1_VDC1] -> bus_selector27/1
  bus_selector28/1 -> bus_creator/29  "<CAN1_WhlSpeed_FL>"
  [R_CAN1_HRW] -> bus_selector28/1
  bus_selector29/1 -> bus_creator/30  "<CAN1_WhlSpeed_FR>"
  [R_CAN1_HRW] -> bus_selector29/1
  bus_selector30/1 -> bus_creator/31  "<CAN1_WhlSpeed_RL>"
  [R_CAN1_HRW] -> bus_selector30/1
  bus_selector31/1 -> bus_creator/32  "<CAN1_WhlSpeed_RR>"
  [R_CAN1_HRW] -> bus_selector31/1
  bus_selector32/1 -> bus_creator/33  "<CAN4_ZFR_CHASSIS_LiningWearFL_Sta>"
  [R_CAN4_ZFR_C5000_0] -> bus_selector32/1
  bus_selector33/1 -> bus_creator/34  "<CAN4_ZFR_CHASSIS_LiningWearFR_Sta>"
  [R_CAN4_ZFR_C5000_0] -> bus_selector33/1
  bus_selector34/1 -> bus_creator/35  "<CAN4_ZRR_CHASSIS_LiningWearRL_Sta>"
  [R_CAN4_ZRR_C5000_0] -> bus_selector34/1
  bus_selector35/1 -> bus_creator/36  "<CAN4_ZRR_CHASSIS_LiningWearRR_Sta>"
  [R_CAN4_ZRR_C5000_0] -> bus_selector35/1
  R_CAN1_AC_BTMS_C5000_0/1 -> [R_CAN1_AC_BTMS_C5000_0]
  R_CAN1_ASC1_A/1 -> [R_CAN1_ASC1_A]
  R_CAN1_EBC1/1 -> [R_CAN1_EBC1]
  R_CAN1_ECAS_DM1/1 -> [R_CAN1_ECAS_DM1]
  R_CAN1_HRW/1 -> [R_CAN1_HRW]
  R_CAN1_TC1/1 -> [R_CAN1_TC1]
  R_CAN1_VDC1/1 -> [R_CAN1_VDC1]
  R_CAN3_B2TM_Info/1 -> [R_CAN3_B2TM_Info]
  R_CAN3_B2V_BattInfo1/1 -> [R_CAN3_B2V_BattInfo1]
  R_CAN3_B2V_ST1/1 -> [R_CAN3_B2V_ST1]
  R_CAN3_B2V_ST2/1 -> [R_CAN3_B2V_ST2]
  R_CAN3_TM_MCUSta2/1 -> [R_CAN3_TM_MCUSta2]
  R_CAN4_ZFR_C100_0/1 -> [R_CAN4_ZFR_C100_0]
  R_CAN4_ZFR_C5000_0/1 -> [R_CAN4_ZFR_C5000_0]
  R_CAN4_ZRR_C5000_0/1 -> [R_CAN4_ZRR_C5000_0]
  R_CAN4_ZRR_CE100_1/1 -> [R_CAN4_ZRR_CE100_1]
  R_CAN4_zGW_CANRr1_C50_0/1 -> [R_CAN4_zGW_CANRr1_C50_0]
